simulink model "total_lab5"  (R2020a)
settings: Solver=VariableStepAuto  StartTime=0.0  StopTime=10.0  RelTol=1e-3
values from neighbouring files (symbols this model uses):
  dZr = 0    [main.m]
  Kd = K_56(i) * M/600/Kt/omega_0    [main.m]
  Ki = Kd*z1*z2    (= 1061.4)    [main.m]
  Kp = Kd*(z1+z2)    (= 1167.54)    [main.m]
  Kt = 3.575e-5    (= 3.575e-05)    [main.m]
  M = 1    [main.m]
  omega_0 = sqrt(G*M/Kt)    [main.m]
  u_0 = omega_0    [main.m]
  w_d = w_d_rpm/60*2*pi    (= 5.23598775598)    [main.m]
  Z0 = 2    [main.m]
settings Model: Creator=josem  LastModifiedBy=josem
settings SolverCC: MaxConsecutiveMinStep=10

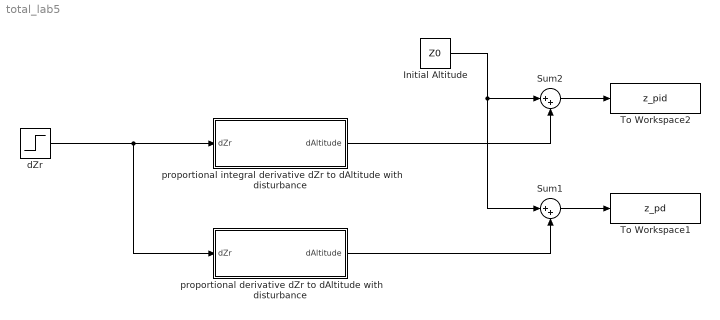
== system total_lab5 ==
  Initial Altitude : Constant  Value=Z0
  Sum1 : Sum  Inputs=|++
  Sum2 : Sum  Inputs=|++
  To Workspace1 : ToWorkspace  VariableName=z_pd  SaveFormat=Structure With Time  SampleTime=-1
  To Workspace2 : ToWorkspace  VariableName=z_pid  SaveFormat=Structure With Time  SampleTime=-1
  dZr : Step  After=dZr  SampleTime=0
  proportional derivative dZr to dAltitude with disturbance : Subsystem
  proportional integral derivative dZr to dAltitude with disturbance : Subsystem
  wires:
  proportional integral derivative dZr to dAltitude with disturbance/1(dAltitude) -> Sum2/2
  Sum2/1 -> To Workspace2/1
  Initial Altitude/1 -> Sum1/1, Sum2/1
  proportional derivative dZr to dAltitude with disturbance/1(dAltitude) -> Sum1/2
  dZr/1 -> proportional derivative dZr to dAltitude with disturbance/1(dZr), proportional integral derivative dZr to dAltitude with disturbance/1(dZr)
  Sum1/1 -> To Workspace1/1

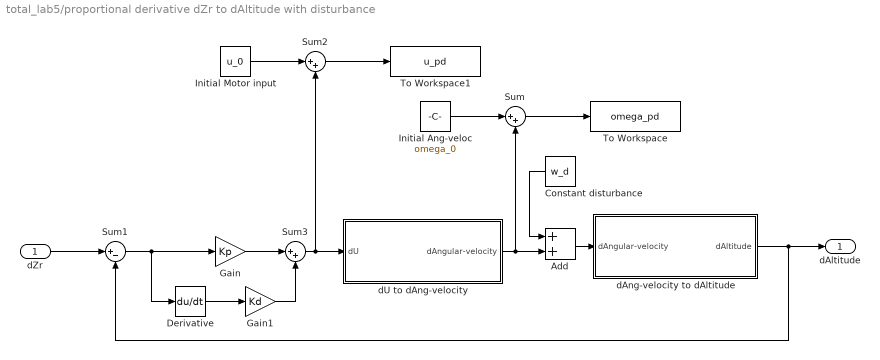
== system total_lab5/proportional derivative dZr to dAltitude with disturbance ==
  dZr : Inport
  Add : Sum
  Constant disturbance : Constant  Value=w_d
  Derivative : Derivative
  Gain : Gain  Gain=Kp
  Gain1 : Gain  Gain=Kd
  Initial Ang-veloc : Constant  Value=omega_0
  Initial Motor input : Constant  Value=u_0
  Sum : Sum  Inputs=|++
  Sum1 : Sum  Inputs=|+-
  Sum2 : Sum  Inputs=|++
  Sum3 : Sum  Inputs=|++
  To Workspace : ToWorkspace  VariableName=omega_pd  SaveFormat=Structure With Time  SampleTime=-1
  To Workspace1 : ToWorkspace  VariableName=u_pd  SaveFormat=Structure With Time  SampleTime=-1
  dAng-velocity to dAltitude : Subsystem
  dU to dAng-velocity : Subsystem
  dAltitude : Outport
  wires:
  dAng-velocity to dAltitude/1(dAltitude) -> Sum1/2, dAltitude/1
  dU to dAng-velocity/1(dAngular-velocity) -> Sum/2, Add/2
  Initial Ang-veloc/1 -> Sum/1
  Sum/1 -> To Workspace/1
  dZr/1 -> Sum1/1
  Sum1/1 -> Derivative/1, Gain/1
  Initial Motor input/1 -> Sum2/1
  Sum2/1 -> To Workspace1/1
  Sum3/1 -> Sum2/2, dU to dAng-velocity/1(dU)
  Gain/1 -> Sum3/1
  Derivative/1 -> Gain1/1
  Gain1/1 -> Sum3/2
  Constant disturbance/1 -> Add/1
  Add/1 -> dAng-velocity to dAltitude/1(dAngular-velocity)

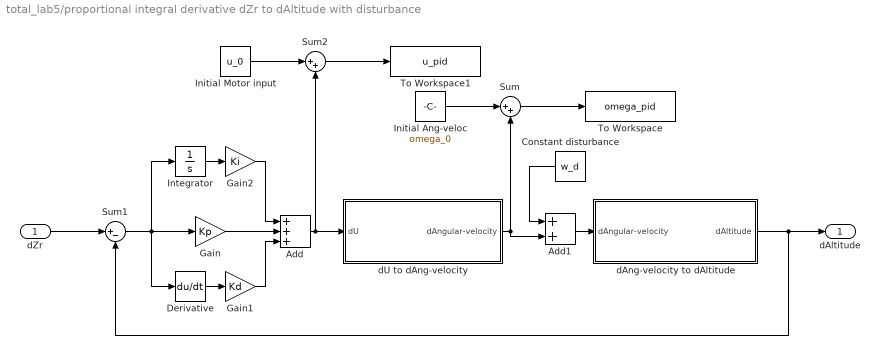
== system total_lab5/proportional integral derivative dZr to dAltitude with disturbance ==
  dZr : Inport
  Add : Sum  Inputs=+++
  Add1 : Sum
  Constant disturbance : Constant  Value=w_d
  Derivative : Derivative
  Gain : Gain  Gain=Kp
  Gain1 : Gain  Gain=Kd
  Gain2 : Gain  Gain=Ki
  Initial Ang-veloc : Constant  Value=omega_0
  Initial Motor input : Constant  Value=u_0
  Integrator : Integrator
  Sum : Sum  Inputs=|++
  Sum1 : Sum  Inputs=|+-
  Sum2 : Sum  Inputs=|++
  To Workspace : ToWorkspace  VariableName=omega_pid  SaveFormat=Structure With Time  SampleTime=-1
  To Workspace1 : ToWorkspace  VariableName=u_pid  SaveFormat=Structure With Time  SampleTime=-1
  dAng-velocity to dAltitude : Subsystem
  dU to dAng-velocity : Subsystem
  dAltitude : Outport
  wires:
  dAng-velocity to dAltitude/1(dAltitude) -> Sum1/2, dAltitude/1
  dU to dAng-velocity/1(dAngular-velocity) -> Add1/2, Sum/2
  Initial Ang-veloc/1 -> Sum/1
  Sum/1 -> To Workspace/1
  dZr/1 -> Sum1/1
  Sum1/1 -> Integrator/1, Gain/1, Derivative/1
  Initial Motor input/1 -> Sum2/1
  Sum2/1 -> To Workspace1/1
  Add/1 -> dU to dAng-velocity/1(dU), Sum2/2
  Derivative/1 -> Gain1/1
  Integrator/1 -> Gain2/1
  Gain1/1 -> Add/3
  Gain/1 -> Add/2
  Gain2/1 -> Add/1
  Constant disturbance/1 -> Add1/1
  Add1/1 -> dAng-velocity to dAltitude/1(dAngular-velocity)

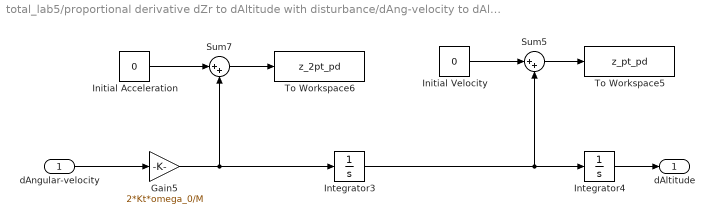
== system total_lab5/proportional derivative dZr to dAltitude with disturbance/dAng-velocity to dAltitude ==
  dAngular-velocity : Inport
  Gain5 : Gain  Gain=2*Kt*omega_0/M
  Initial Acceleration : Constant  Value=0
  Initial Velocity : Constant  Value=0
  Integrator3 : Integrator
  Integrator4 : Integrator
  Sum5 : Sum  Inputs=|++
  Sum7 : Sum  Inputs=|++
  To Workspace5 : ToWorkspace  VariableName=z_pt_pd  SaveFormat=Structure With Time  SampleTime=-1
  To Workspace6 : ToWorkspace  VariableName=z_2pt_pd  SaveFormat=Structure With Time  SampleTime=-1
  dAltitude : Outport
  wires:
  Initial Velocity/1 -> Sum5/1
  Initial Acceleration/1 -> Sum7/1
  Integrator3/1 -> Integrator4/1, Sum5/2
  Sum5/1 -> To Workspace5/1
  Integrator4/1 -> dAltitude/1
  Sum7/1 -> To Workspace6/1
  Gain5/1 -> Integrator3/1, Sum7/2
  dAngular-velocity/1 -> Gain5/1

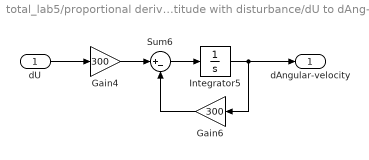
== system total_lab5/proportional derivative dZr to dAltitude with disturbance/dU to dAng-velocity ==
  dU : Inport
  Gain4 : Gain  Gain=300
  Gain6 : Gain  Gain=300
  Integrator5 : Integrator
  Sum6 : Sum  Inputs=|+-
  dAngular-velocity : Outport
  wires:
  Gain4/1 -> Sum6/1
  Gain6/1 -> Sum6/2
  Integrator5/1 -> dAngular-velocity/1, Gain6/1
  Sum6/1 -> Integrator5/1
  dU/1 -> Gain4/1

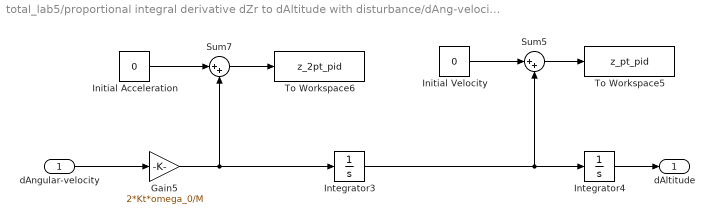
== system total_lab5/proportional integral derivative dZr to dAltitude with disturbance/dAng-velocity to dAltitude ==
  dAngular-velocity : Inport
  Gain5 : Gain  Gain=2*Kt*omega_0/M
  Initial Acceleration : Constant  Value=0
  Initial Velocity : Constant  Value=0
  Integrator3 : Integrator
  Integrator4 : Integrator
  Sum5 : Sum  Inputs=|++
  Sum7 : Sum  Inputs=|++
  To Workspace5 : ToWorkspace  VariableName=z_pt_pid  SaveFormat=Structure With Time  SampleTime=-1
  To Workspace6 : ToWorkspace  VariableName=z_2pt_pid  SaveFormat=Structure With Time  SampleTime=-1
  dAltitude : Outport
  wires:
  Initial Velocity/1 -> Sum5/1
  Initial Acceleration/1 -> Sum7/1
  Integrator3/1 -> Integrator4/1, Sum5/2
  Sum5/1 -> To Workspace5/1
  Integrator4/1 -> dAltitude/1
  Sum7/1 -> To Workspace6/1
  Gain5/1 -> Integrator3/1, Sum7/2
  dAngular-velocity/1 -> Gain5/1

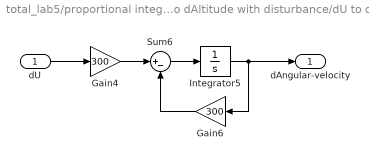
== system total_lab5/proportional integral derivative dZr to dAltitude with disturbance/dU to dAng-velocity ==
  dU : Inport
  Gain4 : Gain  Gain=300
  Gain6 : Gain  Gain=300
  Integrator5 : Integrator
  Sum6 : Sum  Inputs=|+-
  dAngular-velocity : Outport
  wires:
  Gain4/1 -> Sum6/1
  Gain6/1 -> Sum6/2
  Integrator5/1 -> dAngular-velocity/1, Gain6/1
  Sum6/1 -> Integrator5/1
  dU/1 -> Gain4/1
